simulink model "FiboSimulink_RapidAccelerator"  (R2025b)
settings: Solver=FixedStepDiscrete  StartTime=0.0  StopTime=0.9  FixedStep=1  RelTol=1e-3
undefined symbols (not defined in the file or in its folder): n
settings Model: SimulationMode=rapid-accelerator  Creator=marcu  LastModifiedBy=marcu

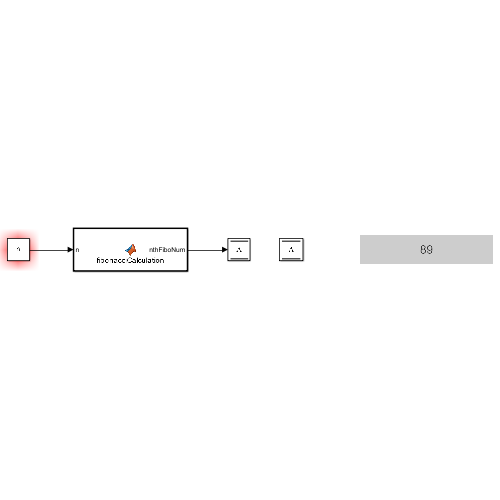
[thumbnail: Simulink's stored preview of the top-level diagram]
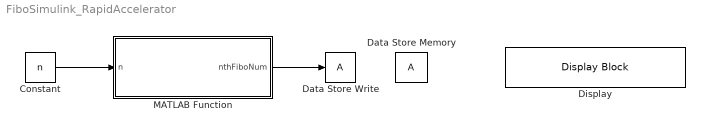
== system FiboSimulink_RapidAccelerator ==
  Constant : Constant  Value=n
  Data Store Memory : DataStoreMemory  WriteAfterWriteMsg=warning  ShowAdditionalParam=off
  Data Store Write : DataStoreWrite  IndexOptions=Index vector (dialog)  Indices=1  OutputSizes=1
  Display : DisplayBlock  LabelPosition=Hide  Transparency=1  GridColor=[0.502, 0.502, 0.502]
  MATLAB Function : MATLAB Function  TreatAsAtomicUnit=on
  wires:
  Constant/1 -> MATLAB Function/1(n)
  MATLAB Function/1(nthFiboNum) -> Data Store Write/1

== matlab function FiboSimulink_RapidAccelerator/MATLAB Function ==
  data: n input; nthFiboNum output
function nthFiboNum = fibonacciCalculation(n)
    arguments
        n (1,1) {mustBeNumeric, mustBeNonnegative, mustBeInteger}
    end

    if n == 0
        nthFiboNum = 0;
        return;
    elseif n == 1
        nthFiboNum = 1;
        return;
    end

    nthFiboNum = fibonacciCalculation(n-1) + fibonacciCalculation(n-2);
end
